simulink model "dspaudioeffects"  (Simulink 8.3)
settings: Solver=FixedStepDiscrete  StartTime=0.0  StopTime=inf  RelTol=1e-3
model workspace (MAT data in the model file):
  x_afxf = [-5.60233913486e-19 -0.0149693400479 -0.00974944717929 0.000149188119263 -0.0143138955012 -0.0134928980062 0.0128597131211 0.0147831216895 0.000166209340046 0.00919720692694 0.0138074287787 -0.0155235118214 ... (86751 elements, 86751x1)]
  fs_afxf = 22050
PreLoadFcn:
  | load dspafxf
libraries: dspsigops x3, dspvision x1, dspsrcs4 x1, dspmisc x1, dspsnks4 x1
settings Model: Creator=The MathWorks Inc.
settings SolverCC: InsertRTBMode=Auto
settings OptimizationCC: ExpressionDepthLimit=2147483647  InitFltsAndDblsToZero=on
settings DebuggingCC: SolverPrmCheckMsg=none  FcnCallInpInsideContextMsg=UseLocalSettings

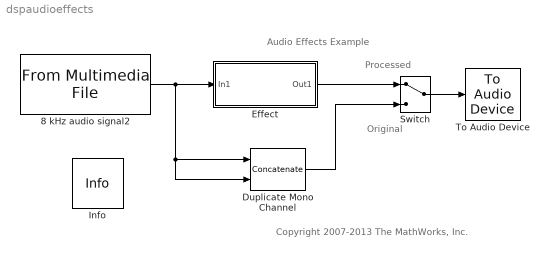
== system dspaudioeffects ==
  note: Audio Effects Example
  note: Original
  note: Processed
  note: Copyright 2007-2013 The MathWorks, Inc.
  8 kHz audio signal2 : dspvision/From Multimedia File  inputFilename=dspafxf.wav  loop=on  numPlays=inf  outputStreams=Audio only  videoDataType=single  audioDataType=double  inheritSampleTime=on  userDefinedSampleTime=1/30  noAudioOutput=off  isIntensityVideo=off  fourcc=RGB  colorVideoFormat=Separate color signals  outputEOF=off  dataOrg=Column-major  audioFrameSize=128  computeAudioFrameSize=off  outSamplingMode=Frame based
  Duplicate Mono Channel : Concatenate  Mode=Multidimensional array  ConcatenateDimension=2
  Effect : Subsystem  mask(Audio Effects){effect=Flanging}
      mask prompts: effect "Audio effect"
      mask help: Select an audio effect
      mask init:
      | if effect == 1
      |     str = 'Flanging';
      | elseif effect == 2
      |     str = 'Reverberation';
      | else
      |     str = 'Stereo';  
      | end
      mask TypeOptions effect: Flanging | Reverberation | Stereo
      mask Display: disp(str)
  Info : dspmisc/Info  SystemSampleTime=-1
  Switch : ManualSwitch
  To Audio Device : dspsnks4/To Audio Device  deviceName=Default  inheritSampleRate=on  sampleRate=44100  deviceDatatype=Determine from input data type  autoBufferSize=on  bufferSize=4096  queueDuration=0.2  defaultOutputChannelMapping=on  outputChannelMapping=1
  wires:
  8 kHz audio signal2/1 -> Effect/1(In1), Duplicate Mono Channel/1, Duplicate Mono Channel/2
  Switch/1 -> To Audio Device/1
  Effect/1(Out1) -> Switch/1
  Duplicate Mono Channel/1 -> Switch/2

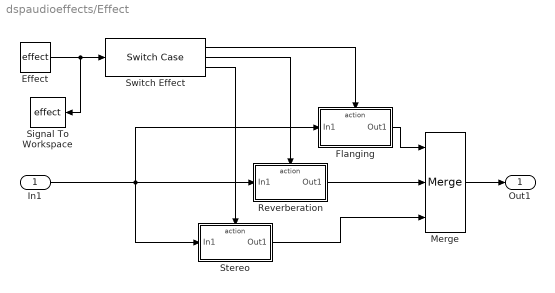
== system dspaudioeffects/Effect ==
  In1 : Inport
  Effect : Constant  Value=effect
  Flanging : Subsystem  TreatAsAtomicUnit=on
  Merge : Merge  Inputs=3
  Reverberation : Subsystem  TreatAsAtomicUnit=on
  Signal To Workspace : ToWorkspace  VariableName=effect  SampleTime=-1
  Stereo : Subsystem  TreatAsAtomicUnit=on
  Switch Effect : SwitchCase  CaseConditions={1,2,3}  ShowDefaultCase=off
  Out1 : Outport
  wires:
  Effect/1 -> Switch Effect/1, Signal To Workspace/1
  Switch Effect/1 -> Flanging/Action
  Switch Effect/2 -> Reverberation/Action
  Switch Effect/3 -> Stereo/Action
  In1/1 -> Reverberation/1(In1), Flanging/1(In1), Stereo/1(In1)
  Reverberation/1(Out1) -> Merge/2
  Merge/1 -> Out1/1
  Flanging/1(Out1) -> Merge/1
  Stereo/1(Out1) -> Merge/3

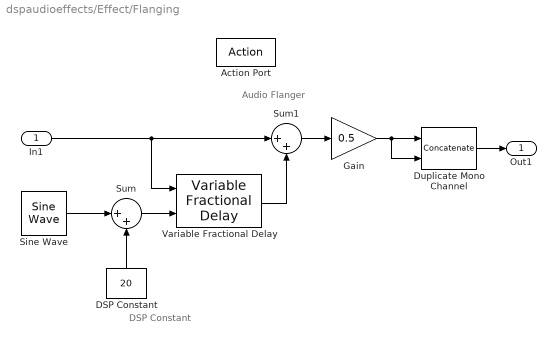
== system dspaudioeffects/Effect/Flanging ==
  note: Audio Flanger
  note: DSP Constant
  In1 : Inport
  Action Port : ActionPort  ActionType=case
  DSP Constant : Constant  Value=20  SampleTime=128/fs_afxf
  Duplicate Mono Channel : Concatenate  Mode=Multidimensional array  ConcatenateDimension=2
  Gain : Gain  Gain=0.5  SaturateOnIntegerOverflow=on  OutDataTypeStr=Inherit: Same as input  ParamDataTypeStr=Inherit: Same as input
  Sine Wave : dspsrcs4/Sine Wave  Amplitude=15  Frequency=1/3.934  Phase=pi/4  SampleMode=Discrete  OutComplex=Real  CompMethod=Trigonometric fcn  TableSize=Speed  SampleTime=1/fs_afxf  SamplesPerFrame=128  ResetState=Restart at time zero  dataType=double  wordLen=16  udDataType=sfix(16)  fracBitsMode=Best precision  numFracBits=15  OutDataTypeStr=double  LastOutDataTypeStr=double
  Sum : Sum  Inputs=|++  SaturateOnIntegerOverflow=on  InputSameDT=on  OutDataTypeStr=Inherit: Same as first input
  Sum1 : Sum  Inputs=|++  SaturateOnIntegerOverflow=on  InputSameDT=on  OutDataTypeStr=Inherit: Same as first input
  Variable Fractional Delay : dspsigops/Variable Fractional Delay  mode=OBSOLETE  modeActive=FIR  dmax=100  InputProcessing=Columns as channels (frame based)  L=8  FarrowL=4  R=10  alpha=0.5  ic=0  fallbackFIR=Switch to linear interpolation if kernel cannot be centered  fallbackFarrow=Clip to the minimum value necessary for centered kernel  noDFT=off  roundingMode=Zero  overflowMode=off
  Out1 : Outport
  wires:
  Sum1/1 -> Gain/1
  Variable Fractional Delay/1 -> Sum1/2
  In1/1 -> Sum1/1, Variable Fractional Delay/1
  Sum/1 -> Variable Fractional Delay/2
  Sine Wave/1 -> Sum/1
  DSP Constant/1 -> Sum/2
  Gain/1 -> Duplicate Mono Channel/1, Duplicate Mono Channel/2
  Duplicate Mono Channel/1 -> Out1/1

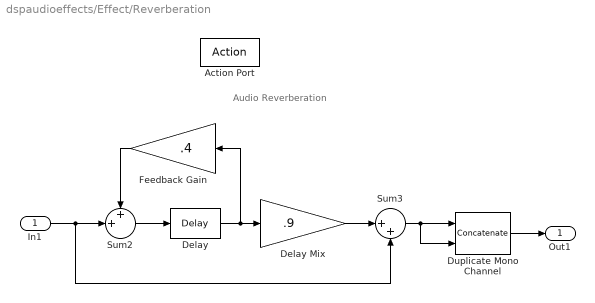
== system dspaudioeffects/Effect/Reverberation ==
  note: Audio Reverberation
  In1 : Inport
  Action Port : ActionPort  ActionType=case
  Delay : dspsigops/Delay  InputProcessing=Columns as channels (frame based)  dly_unit=Samples  delay=1100  ic_detail=on  dif_ic_for_ch=off  dif_ic_for_dly=off  ic=0  reset_popup=None
  Delay Mix : Gain  Gain=.9  SaturateOnIntegerOverflow=on  OutDataTypeStr=Inherit: Same as input  ParamDataTypeStr=Inherit: Same as input
  Duplicate Mono Channel : Concatenate  Mode=Multidimensional array  ConcatenateDimension=2
  Feedback Gain : Gain  Gain=.4  SaturateOnIntegerOverflow=on  OutDataTypeStr=Inherit: Same as input  ParamDataTypeStr=Inherit: Same as input
  Sum2 : Sum  Inputs=++|  SaturateOnIntegerOverflow=on  InputSameDT=on  OutDataTypeStr=Inherit: Same as first input
  Sum3 : Sum  Inputs=|++  SaturateOnIntegerOverflow=on  InputSameDT=on  OutDataTypeStr=Inherit: Same as first input
  Out1 : Outport
  wires:
  In1/1 -> Sum2/2, Sum3/2
  Sum2/1 -> Delay/1
  Feedback Gain/1 -> Sum2/1
  Delay/1 -> Delay Mix/1, Feedback Gain/1
  Delay Mix/1 -> Sum3/1
  Sum3/1 -> Duplicate Mono Channel/1, Duplicate Mono Channel/2
  Duplicate Mono Channel/1 -> Out1/1

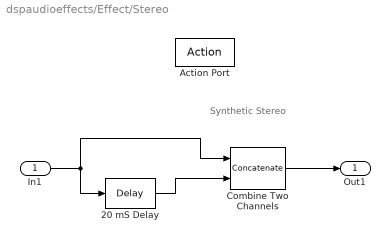
== system dspaudioeffects/Effect/Stereo ==
  note: Synthetic Stereo
  In1 : Inport
  Action Port : ActionPort  ActionType=case
  20 mS Delay : dspsigops/Delay  InputProcessing=Columns as channels (frame based)  dly_unit=Samples  delay=20e-3 * 16000  ic_detail=on  dif_ic_for_ch=off  dif_ic_for_dly=off  ic=0  reset_popup=None
  Combine Two Channels : Concatenate  Mode=Multidimensional array  ConcatenateDimension=2
  Out1 : Outport
  wires:
  20 mS Delay/1 -> Combine Two Channels/2
  In1/1 -> Combine Two Channels/1, 20 mS Delay/1
  Combine Two Channels/1 -> Out1/1
